simulink model "comunicacion"  (R2013a)
settings: Solver=ode3  StartTime=0.0  StopTime=60000  FixedStep=0.01  RelTol=0.5e-3
undefined symbols (not defined in the file or in its folder): CR, matlabfile
libraries: amg_usbconverter_n_connect_lib x2
settings Model: Creator=Juan Esteban  LastModifiedBy=Juan Esteban

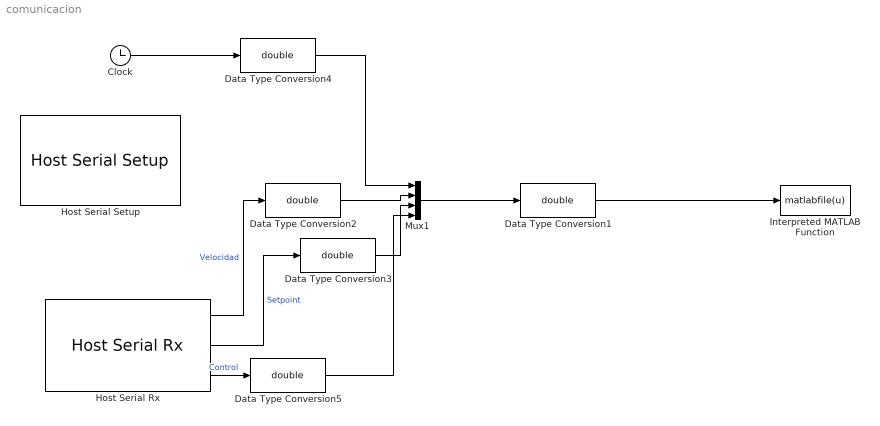
== system comunicacion ==
  Clock : Clock
  Data Type Conversion{1..5} (5 alike) : DataTypeConversion  OutDataTypeStr=double
  Host Serial Rx : amg_usbconverter_n_connect_lib/Host Serial Rx  conf=rx  port=<auto>  baudrate=115200  databits=8  parity=None  stopbit=1  flowcontrol=None  transfer=Blocking  timeout=10  packetmode=Ascii  enableinitialvalues=off  initialvalues=[]  binheader='7E 7E'  binterminator='03 03'  porttype_double=0  porttype_single=0  porttype_int8=0  porttype_uint8=0  porttype_int16=0  porttype_uint16=0  porttype_int32=0  porttype_uint32=2  asciiformat='%f,%f,%f'  rx_asciiterminator="CR (0x0D - \"\\r\")"  tx_asciiterminator="CRLF (0x0D 0x0A - \"\\r\\n\")"  sampletime=-1  enablecustomportlabel=off  cinputportlabel=0  coutputportlabel=A  portpinstr=0  blockid=HostSerialRx  inputporttype=[]  inputportwidth=[]  inputportlabel={}  outputporttype=[1 1 1]  outputportwidth=[1 1 1]  outputportlabel={'(single) %f','(single) %f','(single) %f'}  compat=0  optionstring=[]  autoport='COM8'
  Host Serial Setup : amg_usbconverter_n_connect_lib/Host Serial Setup  conf=setup  port=<auto>  baudrate=115200  databits=8  parity=None  stopbit=1  flowcontrol=None  transfer=Blocking  timeout=2  packetmode=Binary  initialvalues=[]  binheader='7E 7E'  binterminator='03 03'  porttype_double=0  porttype_single=1  porttype_int8=0  porttype_uint8=0  porttype_int16=0  porttype_uint16=0  porttype_int32=0  porttype_uint32=2  asciiformat='%d %u %x'  rx_asciiterminator="CRLF (0x0D 0x0A - \"\\r\\n\")"  tx_asciiterminator="CRLF (0x0D 0x0A - \"\\r\\n\")"  sampletime=-1  enablecustomportlabel=off  cinputportlabel=0  coutputportlabel=A  portpinstr=0  blockid=HostSerialSetup  inputporttype=[]  inputportwidth=[]  inputportlabel={}  outputporttype=[]  outputportwidth=[]  outputportlabel={}  compat=0  optionstring=[]  autoport='COM8'
  Interpreted MATLAB Function : MATLABFcn  MATLABFcn=matlabfile(u)  OutputDimensions=0
  Mux1 : Mux
  wires:
  Host Serial Rx/2 -> Data Type Conversion3/1  "Setpoint"
  Host Serial Rx/1 -> Data Type Conversion2/1  "Velocidad"
  Mux1/1 -> Data Type Conversion1/1
  Clock/1 -> Data Type Conversion4/1
  Data Type Conversion1/1 -> Interpreted MATLAB Function/1
  Data Type Conversion2/1 -> Mux1/2
  Data Type Conversion3/1 -> Mux1/3
  Data Type Conversion4/1 -> Mux1/1
  Host Serial Rx/3 -> Data Type Conversion5/1  "Control"
  Data Type Conversion5/1 -> Mux1/4
